simulink model "be1"  (R2013a)
settings: Solver=ode45  StartTime=0.0  StopTime=10.0  RelTol=1e-3
values from neighbouring files (symbols this model uses):
  Borne_saturation = Valim    (= 35)    [variablesCC.m]
  f0 = 4.2*10^(-4)    (= 0.00042)    [variablesCC.m]
  f1 = 1.5 * 10^(-4)    (= 0.00015)    [variablesCC.m]
  H = 0.2    [variablesCC.m]
  Iref = 2    [variablesCC.m]
  J = 9.2 * 10^(-5)    (= 9.2e-05)    [variablesCC.m]
  Kfem = 60 * 10^(-3)    (= 0.06)    [variablesCC.m]
  Kic = L*wbpc    [variablesCC.m]
  Km = 60 * 10^(-3)    (= 0.06)    [variablesCC.m]
  L = 2.3 * 10 ^(-3)    (= 0.0023)    [variablesCC.m]
  R = 1.2    [variablesCC.m]
  Td = 250 * 10^(-6)    (= 0.00025)    [variablesCC.m]
  Tic = (sqrt(10))/wbpc    [variablesCC.m]
  Valim = 35    [variablesCC.m]
libraries: simulink x1
settings Model: Creator=tfumey  LastModifiedBy=tfumey
settings DebuggingCC: MaxConsecutiveZCsMsg=none

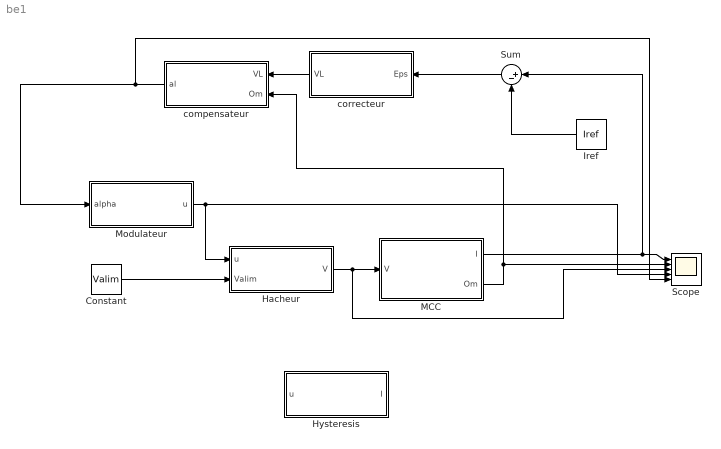
== system be1 ==
  Constant : Constant  Value=Valim
  Hacheur : Subsystem
  Hysteresis : Subsystem
  Iref : Constant  Value=Iref
  MCC : Subsystem
  Modulateur : Subsystem
  Scope : Scope  NumInputPorts=5
      settings: YMin=-3.2~-266.37~-35~0~0.228297  YMax=-1.8~-266.345~35~1~0.228317
  Sum : Sum  Inputs=|+-
  compensateur : Subsystem
  correcteur : Subsystem
  wires:
  MCC/1(I) -> Sum/1, Scope/1
  MCC/2(Om) -> Scope/2, compensateur/2(Om)
  Hacheur/1(V) -> Scope/3, MCC/1(V)
  Constant/1 -> Hacheur/2(Valim)
  Modulateur/1(u) -> Scope/4, Hacheur/1(u)
  correcteur/1(VL) -> compensateur/1(VL)
  compensateur/1("al ") -> Scope/5, Modulateur/1("alpha ")
  Sum/1 -> correcteur/1(Eps)
  Iref/1 -> Sum/2

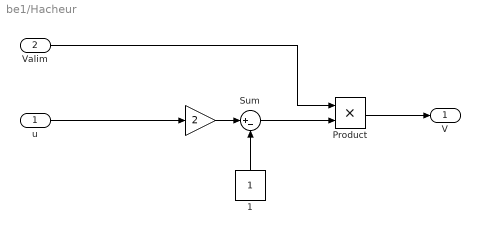
== system be1/Hacheur ==
  u : Inport
  Valim : Inport  Port=2
  " " : Gain  Gain=2
  1 : Constant
  Product : Product
  Sum : Sum  Inputs=|+-
  V : Outport
  wires:
  u/1 -> " "/1
  " "/1 -> Sum/1
  1/1 -> Sum/2
  Sum/1 -> Product/2
  Valim/1 -> Product/1
  Product/1 -> V/1

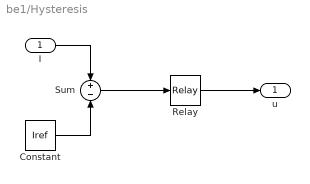
== system be1/Hysteresis ==
  I : Inport
  Constant : Constant  Value=Iref
  Relay : Relay  OnSwitchValue=H  OffSwitchValue=-H  OnOutputValue=0  OffOutputValue=1
  Sum : Sum  Inputs=+|-
  u : Outport
  wires:
  I/1 -> Sum/1
  Relay/1 -> u/1
  Constant/1 -> Sum/2
  Sum/1 -> Relay/1

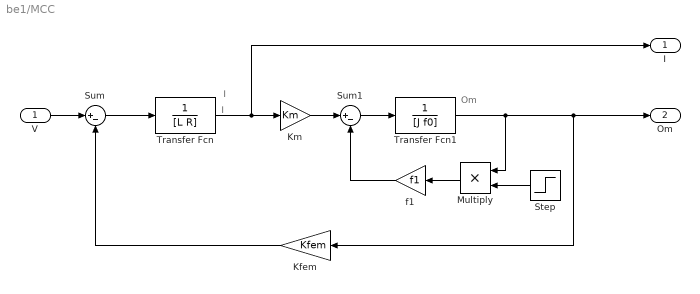
== system be1/MCC ==
  note: I
  note: I
  note: Om
  V : Inport
  Kfem : Gain  Gain=Kfem
  Km : Gain  Gain=Km
  Multiply : Product  Inputs=**
  Step : Step  Time=0.1  SampleTime=0
  Sum : Sum  Inputs=|+-
  Sum1 : Sum  Inputs=|+-
  Transfer Fcn : TransferFcn  Denominator=[L R]
  Transfer Fcn1 : TransferFcn  Denominator=[J f0]
  f1 : Gain  Gain=f1
  I : Outport
  Om : Outport  Port=2
  wires:
  V/1 -> Sum/1
  Kfem/1 -> Sum/2
  Sum/1 -> Transfer Fcn/1
  Transfer Fcn/1 -> I/1, Km/1
  Transfer Fcn1/1 -> Multiply/1, Om/1, Kfem/1
  Sum1/1 -> Transfer Fcn1/1
  Km/1 -> Sum1/1
  f1/1 -> Sum1/2
  Multiply/1 -> f1/1
  Step/1 -> Multiply/2

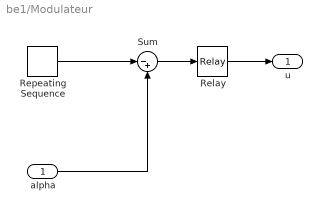
== system be1/Modulateur ==
  "alpha " : Inport
  Relay : Relay
  Repeating Sequence : simulink/Sources/Repeating Sequence  rep_seq_t=[0 Td]  rep_seq_y=[0 1]
  Sum : Sum  Inputs=|-+
  u : Outport
  wires:
  Repeating Sequence/1 -> Sum/1
  "alpha "/1 -> Sum/2
  Sum/1 -> Relay/1
  Relay/1 -> u/1

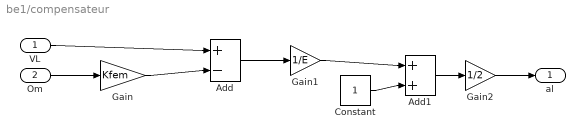
== system be1/compensateur ==
  VL : Inport
  Om : Inport  Port=2
  Add : Sum  Inputs=+||-
  Add1 : Sum  Inputs=+||+
  Constant : Constant
  Gain : Gain  Gain=Kfem
  Gain1 : Gain  Gain=1/E
  Gain2 : Gain  Gain=1/2
  "al " : Outport
  wires:
  Gain/1 -> Add/2
  Om/1 -> Gain/1
  VL/1 -> Add/1
  Add/1 -> Gain1/1
  Gain1/1 -> Add1/1
  Constant/1 -> Add1/2
  Add1/1 -> Gain2/1
  Gain2/1 -> "al "/1

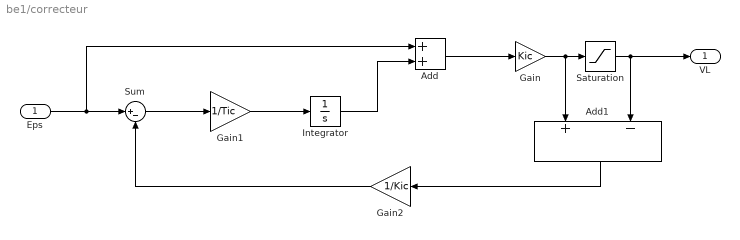
== system be1/correcteur ==
  Eps : Inport
  Add : Sum
  Add1 : Sum  Inputs=+-
  Gain : Gain  Gain=Kic
  Gain1 : Gain  Gain=1/Tic
  Gain2 : Gain  Gain=1/Kic
  Integrator : Integrator
  Saturation : Saturate  UpperLimit=Borne_saturation  LowerLimit=-Borne_saturation
  Sum : Sum  Inputs=|+-
  VL : Outport
  wires:
  Eps/1 -> Add/1, Sum/1
  Gain2/1 -> Sum/2
  Add1/1 -> Gain2/1
  Gain1/1 -> Integrator/1
  Sum/1 -> Gain1/1
  Integrator/1 -> Add/2
  Add/1 -> Gain/1
  Gain/1 -> Saturation/1, Add1/1
  Saturation/1 -> Add1/2, VL/1
